simulink model "quad_mpc_nn"  (R2020a)
settings: Solver=FixedStepAuto  StartTime=0.0  StopTime=20  FixedStep=0.01  RelTol=1e-3
values from neighbouring files (symbols this model uses):
  no_y = 12    [main_quad_mpc.m]
  x0 = [7;-10;0;0;0;0;0;0;0;0;0;0]    [main_quad_mpc.m]
libraries: neural x55
(part 1 of 3)
settings Model: Creator=kekatos  LastModifiedBy=kekatos
settings DebuggingCC: UnderSpecifiedDimensionMsg=warning

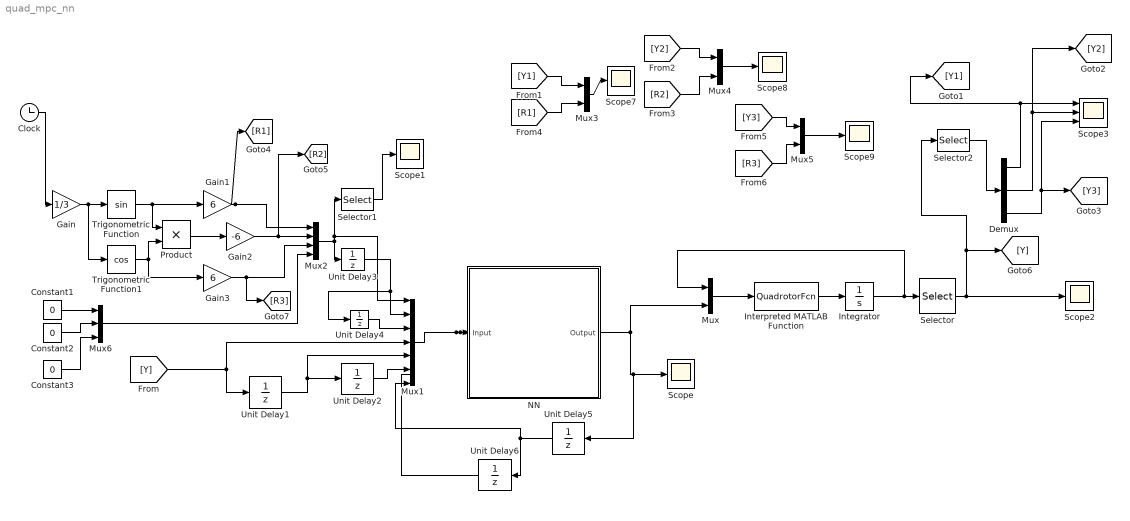
== system quad_mpc_nn ==
  Clock : Clock
  Constant1 : Constant  Value=0
  Constant2 : Constant  Value=0
  Constant3 : Constant  Value=0
  Demux : Demux  Outputs=3
  Gain : Gain  Gain=1/3
  Gain1 : Gain  Gain=6
  Gain2 : Gain  Gain=-6
  Gain3 : Gain  Gain=6
  Integrator : Integrator  InitialCondition=x0
  Interpreted MATLAB Function : MATLABFcn  MATLABFcn=QuadrotorFcn  OutputDimensions=12
  Mux{,3..5} (4 alike) : Mux  Inputs=2
  Mux1 : Mux  Inputs=7
  Mux2 : Mux
  Mux6 : Mux  Inputs=3
  NN : Subsystem
      mask help: Feed-Forward Neural Network
      mask Display: e = 0.06;c1 = [120 150 230]/255;c2 = ([120 150 230]+0)/383;c3 = ([120 150 230]+128)/383;patch([0 1 1 0],[0 0 1 1],c1);patch([0 1 1 1-e 1-e 0+e],[0 0 1 1-e 0+e 0+e],c2);patch([0 0 1 1-e 0+e 0+e],[0 1 1 1-e 1-e 0+e],c3);plot([0 1 1 0 0],[0 0 1 1 0]);fprintf('NNET');port_label('input',1,' Input');port_label('output',1,'Output ');
  Product : Product
  Scope{,1..2,7..9} (6 alike) : Scope
  Scope3 : Scope  NumInputPorts=3
  Selector : Selector  InputPortWidth=12  IndexOptions=Index vector (dialog)  Indices=[1:no_y]  OutputSizes=1
  Selector1 : Selector  InputPortWidth=6  IndexOptions=Index vector (dialog)  Indices=[1:3]  OutputSizes=1
  Selector2 : Selector  InputPortWidth=12  IndexOptions=Index vector (dialog)  Indices=[1:3]  OutputSizes=1
  Trigonometric Function : Trigonometry
  Trigonometric Function1 : Trigonometry  Operator=cos
  Unit Delay{1..6} (6 alike) : UnitDelay  SampleTime=-1  HasFrameUpgradeWarning=on
  wires:
  NN/1(Output) -> Mux/2, Unit Delay5/1, Scope/1
  Interpreted MATLAB Function/1 -> Integrator/1
  Demux/3 -> Scope3/3, [Y3]
  Demux/1 -> [Y1], Scope3/1
  Demux/2 -> [Y2], Scope3/2
  Clock/1 -> Gain/1
  Gain/1 -> Trigonometric Function1/1, Trigonometric Function/1
  Trigonometric Function/1 -> Product/1, Gain1/1
  Trigonometric Function1/1 -> Gain3/1, Product/2
  Product/1 -> Gain2/1
  Gain1/1 -> Mux2/1, [R1]
  Gain2/1 -> [R2], Mux2/2
  Gain3/1 -> Mux2/3, [R3]
  Mux2/1 -> Selector1/1, Mux1/1, Unit Delay3/1
  [Y] -> Mux1/4, Unit Delay1/1
  Mux/1 -> Interpreted MATLAB Function/1
  [Y1] -> Mux3/1
  [R1] -> Mux3/2
  [Y2] -> Mux4/1
  [R2] -> Mux4/2
  [R3] -> Mux5/2
  [Y3] -> Mux5/1
  Mux3/1 -> Scope7/1
  Mux4/1 -> Scope8/1
  Mux5/1 -> Scope9/1
  Integrator/1 -> Mux/1, Selector/1
  Selector/1 -> Selector2/1, [Y], Scope2/1
  Unit Delay1/1 -> Mux1/5, Unit Delay2/1
  Unit Delay3/1 -> Unit Delay4/1, Mux1/2
  Mux1/1 -> NN/1(Input)
  Unit Delay5/1 -> Unit Delay6/1, Mux1/7
  Unit Delay6/1 -> ?
  Constant1/1 -> Mux6/1
  Constant3/1 -> Mux6/3
  Constant2/1 -> Mux6/2
  Unit Delay2/1 -> Mux1/6
  Unit Delay4/1 -> Mux1/3
  Mux6/1 -> Mux2/4
  Selector1/1 -> Scope1/1
  Selector2/1 -> Demux/1

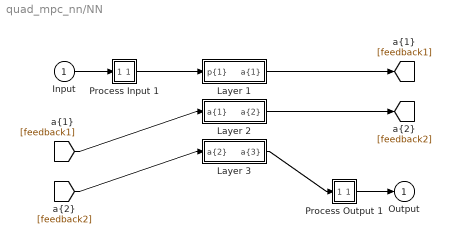
== system quad_mpc_nn/NN ==
  Input : Inport  PortDimensions=58
      mask Display: e = 0.06;c1 = [120 230 180]/255;c2 = ([120 230 180]+0)/(256+128);c3 = ([120 230 180]+128)/(256+128);patch([0 1 1 0],[0 0 1 1],c1);patch([0 1 1 1-e 1-e 0+e],[0 0 1 1-e 0+e 0+e],c2);patch([0 0 1 1-e 0+e 0+e],[0 1 1 1-e 1-e 0+e],c3);plot([0 1 1 0 0],[0 0 1 1 0]);
  Layer 1 : Subsystem
      mask Display: e = 0.06;c1 = [120 150 230]/255;c2 = ([120 150 230]+0)/383;c3 = ([120 150 230]+128)/383;patch([0 1 1 0],[0 0 1 1],c1);patch([0 1 1 1-e 1-e 0+e],[0 0 1 1-e 0+e 0+e],c2);patch([0 0 1 1-e 0+e 0+e],[0 1 1 1-e 1-e 0+e],c3);plot([0 1 1 0 0],[0 0 1 1 0]);
  Layer 2 : Subsystem
      mask Display: e = 0.06;c1 = [120 150 230]/255;c2 = ([120 150 230]+0)/383;c3 = ([120 150 230]+128)/383;patch([0 1 1 0],[0 0 1 1],c1);patch([0 1 1 1-e 1-e 0+e],[0 0 1 1-e 0+e 0+e],c2);patch([0 0 1 1-e 0+e 0+e],[0 1 1 1-e 1-e 0+e],c3);plot([0 1 1 0 0],[0 0 1 1 0]);
  Layer 3 : Subsystem
      mask Display: e = 0.06;c1 = [120 150 230]/255;c2 = ([120 150 230]+0)/383;c3 = ([120 150 230]+128)/383;patch([0 1 1 0],[0 0 1 1],c1);patch([0 1 1 1-e 1-e 0+e],[0 0 1 1-e 0+e 0+e],c2);patch([0 0 1 1-e 0+e 0+e],[0 1 1 1-e 1-e 0+e],c3);plot([0 1 1 0 0],[0 0 1 1 0]);
  Process Input 1 : Subsystem
      mask Display: e = 0.06;c1 = [120 150 230]/255;c2 = ([120 150 230]+0)/383;c3 = ([120 150 230]+128)/383;patch([0 1 1 0],[0 0 1 1],c1);patch([0 1 1 1-e 1-e 0+e],[0 0 1 1-e 0+e 0+e],c2);patch([0 0 1 1-e 0+e 0+e],[0 1 1 1-e 1-e 0+e],c3);plot([0 1 1 0 0],[0 0 1 1 0]);
  Process Output 1 : Subsystem
      mask Display: e = 0.06;c1 = [120 150 230]/255;c2 = ([120 150 230]+0)/383;c3 = ([120 150 230]+128)/383;patch([0 1 1 0],[0 0 1 1],c1);patch([0 1 1 1-e 1-e 0+e],[0 0 1 1-e 0+e 0+e],c2);patch([0 0 1 1-e 0+e 0+e],[0 1 1 1-e 1-e 0+e],c3);plot([0 1 1 0 0],[0 0 1 1 0]);
  Output : Outport  InitialOutput=[0;0;0;0]
      mask Display: e = 0.06;c1 = [120 230 180]/255;c2 = ([120 230 180]+0)/(256+128);c3 = ([120 230 180]+128)/(256+128);patch([0 1 1 0],[0 0 1 1],c1);patch([0 1 1 1-e 1-e 0+e],[0 0 1 1-e 0+e 0+e],c2);patch([0 0 1 1-e 0+e 0+e],[0 1 1 1-e 1-e 0+e],c3);plot([0 1 1 0 0],[0 0 1 1 0]);
  wires:
  Input/1 -> Process Input 1/1(x)
  Process Output 1/1(y) -> Output/1
  Process Input 1/1(p) -> Layer 1/1("p{1}")
  Layer 1/1("a{1}") -> [feedback1]
  [feedback1] -> Layer 2/1("a{1} ")
  Layer 2/1("a{2}") -> [feedback2]
  [feedback2] -> Layer 3/1("a{2} ")
  Layer 3/1("a{3}") -> Process Output 1/1(a)

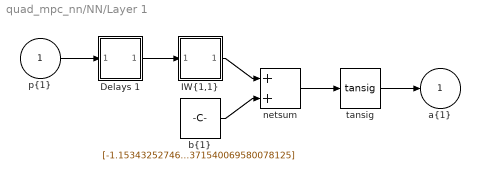
== system quad_mpc_nn/NN/Layer 1 ==
  "p{1}" : Inport  PortDimensions=49
      mask Display: e = 0.06;c1 = [120 230 180]/255;c2 = ([120 230 180]+0)/(256+128);c3 = ([120 230 180]+128)/(256+128);patch([0 1 1 0],[0 0 1 1],c1);patch([0 1 1 1-e 1-e 0+e],[0 0 1 1-e 0+e 0+e],c2);patch([0 0 1 1-e 0+e 0+e],[0 1 1 1-e 1-e 0+e],c3);plot([0 1 1 0 0],[0 0 1 1 0]);
  Delays 1 : Subsystem
      mask Display: e = 0.06;c1 = [120 150 230]/255;c2 = ([120 150 230]+0)/383;c3 = ([120 150 230]+128)/383;patch([0 1 1 0],[0 0 1 1],c1);patch([0 1 1 1-e 1-e 0+e],[0 0 1 1-e 0+e 0+e],c2);patch([0 0 1 1-e 0+e 0+e],[0 1 1 1-e 1-e 0+e],c3);plot([0 1 1 0 0],[0 0 1 1 0]);disp('0');
  "IW{1,1}" : Subsystem
      mask Display: e = 0.06;c1 = [120 150 230]/255;c2 = ([120 150 230]+0)/383;c3 = ([120 150 230]+128)/383;patch([0 1 1 0],[0 0 1 1],c1);patch([0 1 1 1-e 1-e 0+e],[0 0 1 1-e 0+e 0+e],c2);patch([0 0 1 1-e 0+e 0+e],[0 1 1 1-e 1-e 0+e],c3);plot([0 1 1 0 0],[0 0 1 1 0]);disp('W');
  "b{1}" : Constant  Value=[-1.1534325274653685067249853091198019683361053466796875;1.4966260613036046489554564686841331422328948974609375;-1.005683782892233590899877526680938899517059326171875;-0.5585149137775207162093238366651348769664764404296875;0.5156948740228484151515431221923790872097015380859375;0.270652358371207213405540414896677248179912567138671875;-0.58182389607502005279826562400558032095432281494140625;-0.505018414312629726481418401817791163921356201171875;0.06062119703017955496537894077846431173384189605712890625;0.71474409270376659808476915713981725275516510009765625;-0.319936030103037560845535836051567457616329193115234375;0.52080363270864882263566641995566897094249725341796875;-0.292906678892674021685849083951325155794620513916015625;-0.170657115188820485141008020946173928678035736083984375;0.24242229030938045042375961202196776866912841796875;-0.09903380557279552187655013995026820339262485504150390625;0.271407977842606396023938941652886569499969482421875;0.363829208956005623054608122401987202465534210205078125;-0.241764019068507141074775290690013207495212554931640625;-0.44964027937027772896527721968595869839191436767578125;0.70440013311789606564872201488469727337360382080078125;0.31782453909131758162942560375086031854152679443359375;1.031412642847730598560929138329811394214630126953125;0.61399467700719423390864903922192752361297607421875;-0.9756353765460430427225446692318655550479888916015625;1.232363130417662322457772461348213255405426025390625;1.2857310973093183381621429361985065042972564697265625;1.2805238927783320068698458271683193743228912353515625;1.1791045040388510312112657629768364131450653076171875;-1.2433017469216587347347058312152512371540069580078125]
      mask Display: e = 0.06;c1 = [120 150 230]/255;c2 = ([120 150 230]+0)/383;c3 = ([120 150 230]+128)/383;patch([0 1 1 0],[0 0 1 1],c1);patch([0 1 1 1-e 1-e 0+e],[0 0 1 1-e 0+e 0+e],c2);patch([0 0 1 1-e 0+e 0+e],[0 1 1 1-e 1-e 0+e],c3);plot([0 1 1 0 0],[0 0 1 1 0]);disp('b');
  netsum : Sum  Inputs=2  InputSameDT=on  SaturateOnIntegerOverflow=on  OutDataTypeStr=Inherit: Same as first input
      mask Display: e = 0.06;c1 = [120 150 230]/255;c2 = ([120 150 230]+0)/383;c3 = ([120 150 230]+128)/383;patch([0 1 1 0],[0 0 1 1],c1);patch([0 1 1 1-e 1-e 0+e],[0 0 1 1-e 0+e 0+e],c2);patch([0 0 1 1-e 0+e 0+e],[0 1 1 1-e 1-e 0+e],c3);plot([0 1 1 0 0],[0 0 1 1 0]);disp('+');
  tansig : neural/Transfer Functions/tansig
  "a{1}" : Outport  InitialOutput=[0;0;0;0;0;0;0;0;0;0;0;0;0;0;0;0;0;0;0;0;0;0;0;0;0;0;0;0;0;0]
      mask Display: e = 0.06;c1 = [120 230 180]/255;c2 = ([120 230 180]+0)/(256+128);c3 = ([120 230 180]+128)/(256+128);patch([0 1 1 0],[0 0 1 1],c1);patch([0 1 1 1-e 1-e 0+e],[0 0 1 1-e 0+e 0+e],c2);patch([0 0 1 1-e 0+e 0+e],[0 1 1 1-e 1-e 0+e],c3);plot([0 1 1 0 0],[0 0 1 1 0]);
  wires:
  "p{1}"/1 -> Delays 1/1("p{1}")
  Delays 1/1("pd{1,1}") -> "IW{1,1}"/1("pd{1,1}")
  "IW{1,1}"/1("iz{1,1}") -> netsum/1
  "b{1}"/1 -> netsum/2
  netsum/1 -> tansig/1
  tansig/1 -> "a{1}"/1

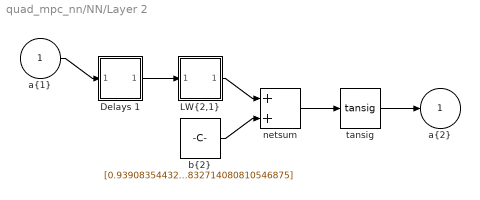
== system quad_mpc_nn/NN/Layer 2 ==
  "a{1} " : Inport  PortDimensions=30
      mask Display: e = 0.06;c1 = [120 230 180]/255;c2 = ([120 230 180]+0)/(256+128);c3 = ([120 230 180]+128)/(256+128);patch([0 1 1 0],[0 0 1 1],c1);patch([0 1 1 1-e 1-e 0+e],[0 0 1 1-e 0+e 0+e],c2);patch([0 0 1 1-e 0+e 0+e],[0 1 1 1-e 1-e 0+e],c3);plot([0 1 1 0 0],[0 0 1 1 0]);
  Delays 1 : Subsystem
      mask Display: e = 0.06;c1 = [120 150 230]/255;c2 = ([120 150 230]+0)/383;c3 = ([120 150 230]+128)/383;patch([0 1 1 0],[0 0 1 1],c1);patch([0 1 1 1-e 1-e 0+e],[0 0 1 1-e 0+e 0+e],c2);patch([0 0 1 1-e 0+e 0+e],[0 1 1 1-e 1-e 0+e],c3);plot([0 1 1 0 0],[0 0 1 1 0]);disp('0');
  "LW{2,1}" : Subsystem
      mask Display: e = 0.06;c1 = [120 150 230]/255;c2 = ([120 150 230]+0)/383;c3 = ([120 150 230]+128)/383;patch([0 1 1 0],[0 0 1 1],c1);patch([0 1 1 1-e 1-e 0+e],[0 0 1 1-e 0+e 0+e],c2);patch([0 0 1 1-e 0+e 0+e],[0 1 1 1-e 1-e 0+e],c3);plot([0 1 1 0 0],[0 0 1 1 0]);disp('W');
  "b{2}" : Constant  Value=[0.9390835443270801885518039853195659816265106201171875;-1.149405163711486377309256567968986928462982177734375;1.3747169047643772454847521657939068973064422607421875;-0.958155417398800057782182193477638065814971923828125;-0.5802168296025504989898990970687009394168853759765625;0.33201081612602123538380283207516185939311981201171875;-0.1776744484559082681851549523344147019088268280029296875;0.165417268974901165989876972162164747714996337890625;-0.51839062848348615997196020543924532830715179443359375;0.2377409149677391086985522861141362227499485015869140625;-0.36941486081352703507718615583144128322601318359375;0.76918702278857675747048006087425164878368377685546875;1.0716349308080890256889006195706315338611602783203125;1.436745794260417152798936513136141002178192138671875;-1.1223522453607397419972357965889386832714080810546875]
      mask Display: e = 0.06;c1 = [120 150 230]/255;c2 = ([120 150 230]+0)/383;c3 = ([120 150 230]+128)/383;patch([0 1 1 0],[0 0 1 1],c1);patch([0 1 1 1-e 1-e 0+e],[0 0 1 1-e 0+e 0+e],c2);patch([0 0 1 1-e 0+e 0+e],[0 1 1 1-e 1-e 0+e],c3);plot([0 1 1 0 0],[0 0 1 1 0]);disp('b');
  netsum : Sum  Inputs=2  InputSameDT=on  SaturateOnIntegerOverflow=on  OutDataTypeStr=Inherit: Same as first input
      mask Display: e = 0.06;c1 = [120 150 230]/255;c2 = ([120 150 230]+0)/383;c3 = ([120 150 230]+128)/383;patch([0 1 1 0],[0 0 1 1],c1);patch([0 1 1 1-e 1-e 0+e],[0 0 1 1-e 0+e 0+e],c2);patch([0 0 1 1-e 0+e 0+e],[0 1 1 1-e 1-e 0+e],c3);plot([0 1 1 0 0],[0 0 1 1 0]);disp('+');
  tansig : neural/Transfer Functions/tansig
  "a{2}" : Outport  InitialOutput=[0;0;0;0;0;0;0;0;0;0;0;0;0;0;0]
      mask Display: e = 0.06;c1 = [120 230 180]/255;c2 = ([120 230 180]+0)/(256+128);c3 = ([120 230 180]+128)/(256+128);patch([0 1 1 0],[0 0 1 1],c1);patch([0 1 1 1-e 1-e 0+e],[0 0 1 1-e 0+e 0+e],c2);patch([0 0 1 1-e 0+e 0+e],[0 1 1 1-e 1-e 0+e],c3);plot([0 1 1 0 0],[0 0 1 1 0]);
  wires:
  "a{1} "/1 -> Delays 1/1("p{2}")
  Delays 1/1("pd{2,1}") -> "LW{2,1}"/1("ad{2,1}")
  "LW{2,1}"/1("lz{2,1}") -> netsum/1
  "b{2}"/1 -> netsum/2
  netsum/1 -> tansig/1
  tansig/1 -> "a{2}"/1

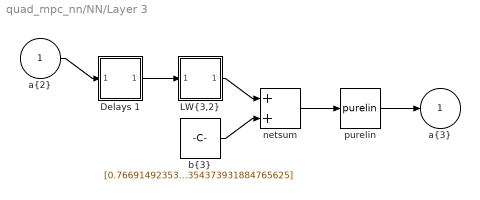
== system quad_mpc_nn/NN/Layer 3 ==
  "a{2} " : Inport  PortDimensions=15
      mask Display: e = 0.06;c1 = [120 230 180]/255;c2 = ([120 230 180]+0)/(256+128);c3 = ([120 230 180]+128)/(256+128);patch([0 1 1 0],[0 0 1 1],c1);patch([0 1 1 1-e 1-e 0+e],[0 0 1 1-e 0+e 0+e],c2);patch([0 0 1 1-e 0+e 0+e],[0 1 1 1-e 1-e 0+e],c3);plot([0 1 1 0 0],[0 0 1 1 0]);
  Delays 1 : Subsystem
      mask Display: e = 0.06;c1 = [120 150 230]/255;c2 = ([120 150 230]+0)/383;c3 = ([120 150 230]+128)/383;patch([0 1 1 0],[0 0 1 1],c1);patch([0 1 1 1-e 1-e 0+e],[0 0 1 1-e 0+e 0+e],c2);patch([0 0 1 1-e 0+e 0+e],[0 1 1 1-e 1-e 0+e],c3);plot([0 1 1 0 0],[0 0 1 1 0]);disp('0');
  "LW{3,2}" : Subsystem
      mask Display: e = 0.06;c1 = [120 150 230]/255;c2 = ([120 150 230]+0)/383;c3 = ([120 150 230]+128)/383;patch([0 1 1 0],[0 0 1 1],c1);patch([0 1 1 1-e 1-e 0+e],[0 0 1 1-e 0+e 0+e],c2);patch([0 0 1 1-e 0+e 0+e],[0 1 1 1-e 1-e 0+e],c3);plot([0 1 1 0 0],[0 0 1 1 0]);disp('W');
  "b{3}" : Constant  Value=[0.7669149235344736581510005635209381580352783203125;0.02981236811184943824581949911589617840945720672607421875;0.45224706500437206191378436415106989443302154541015625;0.63572688067914973064631567467586137354373931884765625]
      mask Display: e = 0.06;c1 = [120 150 230]/255;c2 = ([120 150 230]+0)/383;c3 = ([120 150 230]+128)/383;patch([0 1 1 0],[0 0 1 1],c1);patch([0 1 1 1-e 1-e 0+e],[0 0 1 1-e 0+e 0+e],c2);patch([0 0 1 1-e 0+e 0+e],[0 1 1 1-e 1-e 0+e],c3);plot([0 1 1 0 0],[0 0 1 1 0]);disp('b');
  netsum : Sum  Inputs=2  InputSameDT=on  SaturateOnIntegerOverflow=on  OutDataTypeStr=Inherit: Same as first input
      mask Display: e = 0.06;c1 = [120 150 230]/255;c2 = ([120 150 230]+0)/383;c3 = ([120 150 230]+128)/383;patch([0 1 1 0],[0 0 1 1],c1);patch([0 1 1 1-e 1-e 0+e],[0 0 1 1-e 0+e 0+e],c2);patch([0 0 1 1-e 0+e 0+e],[0 1 1 1-e 1-e 0+e],c3);plot([0 1 1 0 0],[0 0 1 1 0]);disp('+');
  purelin : neural/Transfer Functions/purelin
  "a{3}" : Outport  InitialOutput=[0;0;0;0]
      mask Display: e = 0.06;c1 = [120 230 180]/255;c2 = ([120 230 180]+0)/(256+128);c3 = ([120 230 180]+128)/(256+128);patch([0 1 1 0],[0 0 1 1],c1);patch([0 1 1 1-e 1-e 0+e],[0 0 1 1-e 0+e 0+e],c2);patch([0 0 1 1-e 0+e 0+e],[0 1 1 1-e 1-e 0+e],c3);plot([0 1 1 0 0],[0 0 1 1 0]);
  wires:
  "a{2} "/1 -> Delays 1/1("p{3}")
  Delays 1/1("pd{3,2}") -> "LW{3,2}"/1("ad{3,2}")
  "LW{3,2}"/1("lz{3,2}") -> netsum/1
  "b{3}"/1 -> netsum/2
  netsum/1 -> purelin/1
  purelin/1 -> "a{3}"/1

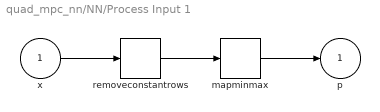
== system quad_mpc_nn/NN/Process Input 1 ==
  x : Inport  PortDimensions=58
      mask Display: e = 0.06;c1 = [120 230 180]/255;c2 = ([120 230 180]+0)/(256+128);c3 = ([120 230 180]+128)/(256+128);patch([0 1 1 0],[0 0 1 1],c1);patch([0 1 1 1-e 1-e 0+e],[0 0 1 1-e 0+e 0+e],c2);patch([0 0 1 1-e 0+e 0+e],[0 1 1 1-e 1-e 0+e],c3);plot([0 1 1 0 0],[0 0 1 1 0]);
  mapminmax : neural/Processing Functions/mapminmax  xmin=[-6.47924894168804232919001151458;-3.20694529587613796905998242437;-6.35280635515283442771305999486;-6.47924894168804232919001151458;-3.20694529587613796905998242437;-6.35280635515283442771305999486;-6.47924894168804232919001151458;-3.20694529587613796905998242437;-6.35280635515283442771305999486;-6.44795089752797156990027360735;-10;-6.32010528970793217240498051979;-1.19063002135584783403032815841;-0.471717602720056361498279784428;-1.66453468285964811812505104172;-4.58645979780001411540979461279;-3.28594363285851631673040174064;-4.78688703022850159385370716336;-1.79000853861525488497363767237;-1.10953386061212277979848295217;-1.41620154255069996551696931419;-6.44795089752797156990027360735;-10;-6.32010528970793217240498051979;-1.19063002135584783403032815841;-0.471717602720056361498279784428;-1.66453468285964811812505104172;-4.58645979780001411540979461279;-3.28594363285851631673040174064;-4.78688703022850159385370716336;-1.79000853861525488497363767237;-1.10953386061212277979848295217;-1.41620154255069996551696931419;-6.44795089752797156990027360735;-10;-6.32010528970793217240498051979;-1.19063002135584783403032815841;-0.471717602720056361498279784428;-1.66453468285964811812505104172;-4.58645979780001411540979461279;-3.28594363285851631673040174064;-4.78688703022850159385370716336;-1.79000853861525488497363767237;-1.10953386061212277979848295217;-1.41620154255069996551696931419;-1.84185682852183363748440106676e-20;-1.3753745846544342886159673695e-20;-1.82664434018961409493581299124e-20;-5.38054982220510749895954017061e-19]  xmax=[6.4796909601784378196498437319;3.20717191846393268050974256766;6.3530230440098041100327463937;6.4796909601784378196498437319;3.20717191846393268050974256766;6.3530230440098041100327463937;6.4796909601784378196498437319;3.20717191846393268050974256766;6.3530230440098041100327463937;8.68411322205773927862537675537;3.62480677837661957596537831705;6.32833054864998967303790777805;0.93647594978114834241011976701;0.602085429619818035540390610549;0.0875271209255244347913205160694;5.69330047648160331164035596885;6.10063101815880237666078755865;6.84099460410426729595201322809;2.43897752470104389743710271432;0.985918743711737266544048452488;0.871527324125089486450690401398;8.68411322205773927862537675537;3.62480677837661957596537831705;6.32833054864998967303790777805;0.93647594978114834241011976701;0.602085429619818035540390610549;0.0875271209255244347913205160694;5.69330047648160331164035596885;6.10063101815880237666078755865;6.84099460410426729595201322809;2.43897752470104389743710271432;0.985918743711737266544048452488;0.871527324125089486450690401398;8.68411322205773927862537675537;3.62480677837661957596537831705;6.32833054864998967303790777805;0.93647594978114834241011976701;0.602085429619818035540390610549;0.0875271209255244347913205160694;5.69330047648160331164035596885;6.10063101815880237666078755865;6.84099460410426729595201322809;2.43897752470104389743710271432;0.985918743711737266544048452488;0.871527324125089486450690401398;12;12;12;12]  ymin=-1  ymax=1
  removeconstantrows : neural/Processing Functions/removeconstantrows  inputSize=58  keep=[1 2 3 7 8 9 13 14 15 19 20 21 22 23 24 25 26 27 28 29 30 31 32 33 34 35 36 37 38 39 40 41 42 43 44 45 46 47 48 49 50 51 52 53 54 55 56 57 58]
      settings: SourceProductBaseCode=NN
  p : Outport  PortDimensions=49
      mask Display: e = 0.06;c1 = [120 230 180]/255;c2 = ([120 230 180]+0)/(256+128);c3 = ([120 230 180]+128)/(256+128);patch([0 1 1 0],[0 0 1 1],c1);patch([0 1 1 1-e 1-e 0+e],[0 0 1 1-e 0+e 0+e],c2);patch([0 0 1 1-e 0+e 0+e],[0 1 1 1-e 1-e 0+e],c3);plot([0 1 1 0 0],[0 0 1 1 0]);
  wires:
  x/1 -> removeconstantrows/1
  removeconstantrows/1 -> mapminmax/1
  mapminmax/1 -> p/1

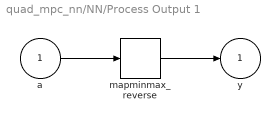
== system quad_mpc_nn/NN/Process Output 1 ==
  a : Inport  PortDimensions=4
      mask Display: e = 0.06;c1 = [120 230 180]/255;c2 = ([120 230 180]+0)/(256+128);c3 = ([120 230 180]+128)/(256+128);patch([0 1 1 0],[0 0 1 1],c1);patch([0 1 1 1-e 1-e 0+e],[0 0 1 1-e 0+e 0+e],c2);patch([0 0 1 1-e 0+e 0+e],[0 1 1 1-e 1-e 0+e],c3);plot([0 1 1 0 0],[0 0 1 1 0]);
  mapminmax_reverse : neural/Processing Functions/mapminmax_reverse  xmin=[-1.84185682852183363748440106676e-20;-1.3753745846544342886159673695e-20;-1.82664434018961409493581299124e-20;-5.38054982220510749895954017061e-19]  xmax=[12;12;12;12]  ymin=-1  ymax=1
  y : Outport  PortDimensions=4
      mask Display: e = 0.06;c1 = [120 230 180]/255;c2 = ([120 230 180]+0)/(256+128);c3 = ([120 230 180]+128)/(256+128);patch([0 1 1 0],[0 0 1 1],c1);patch([0 1 1 1-e 1-e 0+e],[0 0 1 1-e 0+e 0+e],c2);patch([0 0 1 1-e 0+e 0+e],[0 1 1 1-e 1-e 0+e],c3);plot([0 1 1 0 0],[0 0 1 1 0]);
  wires:
  a/1 -> mapminmax_reverse/1
  mapminmax_reverse/1 -> y/1

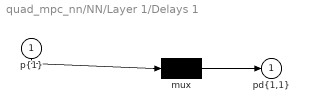
== system quad_mpc_nn/NN/Layer 1/Delays 1 ==
  "p{1}" : Inport  PortDimensions=49
      mask Display: e = 0.06;c1 = [120 230 180]/255;c2 = ([120 230 180]+0)/(256+128);c3 = ([120 230 180]+128)/(256+128);patch([0 1 1 0],[0 0 1 1],c1);patch([0 1 1 1-e 1-e 0+e],[0 0 1 1-e 0+e 0+e],c2);patch([0 0 1 1-e 0+e 0+e],[0 1 1 1-e 1-e 0+e],c3);plot([0 1 1 0 0],[0 0 1 1 0]);
  mux : Mux  Inputs=1
      mask Display: e = 0.06;c1 = [120 150 230]/255;c2 = ([120 150 230]+0)/383;c3 = ([120 150 230]+128)/383;patch([0 1 1 0],[0 0 1 1],c1);patch([0 1 1 1-e 1-e 0+e],[0 0 1 1-e 0+e 0+e],c2);patch([0 0 1 1-e 0+e 0+e],[0 1 1 1-e 1-e 0+e],c3);plot([0 1 1 0 0],[0 0 1 1 0]);disp('Mux')
  "pd{1,1}" : Outport
      mask Display: e = 0.06;c1 = [120 230 180]/255;c2 = ([120 230 180]+0)/(256+128);c3 = ([120 230 180]+128)/(256+128);patch([0 1 1 0],[0 0 1 1],c1);patch([0 1 1 1-e 1-e 0+e],[0 0 1 1-e 0+e 0+e],c2);patch([0 0 1 1-e 0+e 0+e],[0 1 1 1-e 1-e 0+e],c3);plot([0 1 1 0 0],[0 0 1 1 0]);
  wires:
  "p{1}"/1 -> mux/1
  mux/1 -> "pd{1,1}"/1
